simulink model "sop_codegen"  (R2024b)
settings: Solver=FixedStepAuto  StartTime=0.0  StopTime=inf  FixedStep=sopk_stepSize  RelTol=1e-3  SampleTimeConstraint=STIndependent  EnableMultiTasking=on
undefined symbols (not defined in the file): bmsc_CellMaxVolt, bmsc_CellMinVolt, bmsc_InternalChgResistX, bmsc_InternalChgResistY, bmsc_InternalChgResistZ, bmsc_InternalDischgResistX, bmsc_InternalDischgResistY, bmsc_InternalDischgResistZ, bmsc_NumberInPara, bmsc_NumberInSeries, sopc_ChargeDerate, sopc_ChgFaultDerate, sopc_DischargeDerate, sopc_DischgFaultDerate, sopc_SOCVsOCVX, sopc_SOCVsOCVY
settings Model: Creator=favv5g  LastModifiedBy=voillat
settings ConfigSet: Description=OpenECU configuration set for code generation under RTW-EC.
settings SolverCC: AlgebraicLoopSolver=TrustRegion  PositivePriorityOrder=on
settings DataIOCC: LimitDataPoints=on  SaveFormat=Array  SignalLoggingSaveFormat=ModelDataLogs
settings OptimizationCC: DefaultParameterBehavior=Inlined  InlineInvariantSignals=on  ExpressionDepthLimit=2147483647  StateBitsets=on  DataBitsets=on  ZeroExternalMemoryAtStartup=off  ZeroInternalMemoryAtStartup=off  NoFixptDivByZeroProtection=on  EfficientFloat2IntCast=on  LifeSpan=1  EfficientTunableParamExpr=on
settings DebuggingCC: SaveWithParameterizedLinksMsg=none  SignalResolutionControl=TryResolveAllWithWarning  MultiTaskDSMMsg=warning  MultiTaskCondExecSysMsg=none  SingleTaskRateTransMsg=error  CheckMatrixSingularityMsg=warning  VectorMatrixConversionMsg=warning  SignalLabelMismatchMsg=warning  UnconnectedInputMsg=warning  UnconnectedOutputMsg=warning  UnconnectedLineMsg=warning  AllowSymbolicDim=off  StateNameClashWarn=warning  SFUnexpectedBacktrackingDiag=warning  SFNoUnconditionalDefaultTransitionDiag=warning  SFExecutionAtInitializationDiag=none  ArithmeticOperatorsInVariantConditions=warning
settings HardwareCC: ProdBitPerPointer=32  ProdBitPerSizeT=32  ProdBitPerPtrDiffT=32  ProdLargestAtomicInteger=Long  ProdLargestAtomicFloat=Double  ProdEndianess=BigEndian  ProdWordSize=32  ProdHWDeviceType=Freescale->32-bit PowerPC  TargetIntDivRoundTo=Zero  TargetEndianess=BigEndian  TargetHWDeviceType=Freescale->32-bit PowerPC  ProdEqTarget=off
settings ModelReferenceCC: EnableRefExpFcnMdlSchedulingChecks=on  PropagateSignalLabelsOutOfModel=off
settings SFSimCC: SimUseLocalCustomCode=off  MATLABDynamicMemAlloc=off  CustomCodeUndefinedFunction=UseInterfaceOnly
settings RTWCC: Description=OpenECU Platform Target (ERT, optimised floating-point code)  SystemTargetFile=openecu_ert.tlc  MakeCommand=make_rtw optimized_floating_point=1  TemplateMakefile=openecu_ert_r2015b_64.tmf  RetainRTWFile=on  RTWUseLocalCustomCode=off  IncludeHyperlinkInReport=on  GPUComputeCapability=3.5
settings CodeAppCC: ForceParamTrailComments=on  IgnoreCustomStorageClasses=off  SimulinkDataObjDesc=on  CustomSymbolStrType=$N$R$M  InsertBlockDesc=on  StateflowObjectComments=on  InternalIdentifier=Classic
settings STFCustomTargetCC: TargetLibSuffix=.a  GenerateSampleERTMain=on  IncludeMdlTerminateFcn=off  CombineOutputUpdateFcns=on  IncludeFileDelimiter=UseQuote  ERTCustomFileBanners=on  SupportContinuousTime=off  RemoveResetFunc=on  MATLABClassNameForMDSCustomization=Simulink.SoftwareTarget.ERTCustomization  SystemTargetFile=openecu_ert.tlc
settings ERTTargetCC: MultiwordLength=2048  GenerateSampleERTMain=on  ParMdlRefBuildCompliant=off  CompOptLevelCompliant=off  ConcurrentExecutionCompliant=off  IncludeMdlTerminateFcn=off  IncludeFileDelimiter=UseQuote  SupportNonInlinedSFcns=on  ModelStepFunctionPrototypeControlCompliant=off  CPPClassGenCompliant=off  UseToolchainInfoCompliant=off  ExtModeMexFile=noextcomm  ERTSrcFileBannerTemplate=oe_code_c_template.cgt  ERTHdrFileBannerTemplate=oe_code_h_template.cgt  ERTDataSrcFileTemplate=oe_data_c_template.cgt  ERTDataHdrFileTemplate=oe_data_h_template.cgt  ERTCustomFileTemplate=example_file_process.tlc  GlobalDataDefinition=InSeparateSourceFile  GlobalDataReference=InSeparateHeaderFile  ConvertIfToSwitch=off  SuppressUnreachableDefaultCases=off  EnableUserReplacementTypes=on  DynamicArrayContainerType=coder::array
settings ConfigComp: CovMetricSettings=dw  CovSaveCumulativeToWorkspaceVar=on  CovSaveSingleToWorkspaceVar=on  CovExternalEMLEnable=off

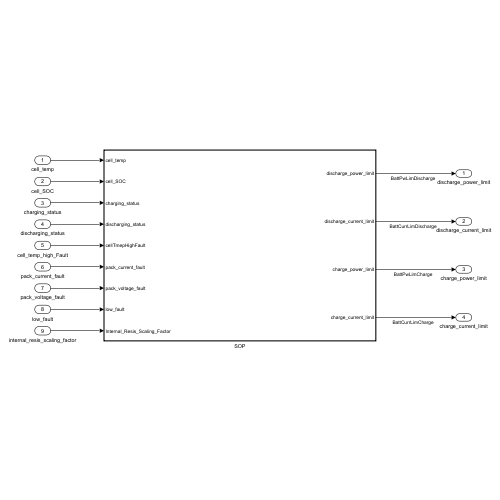
[thumbnail: Simulink's stored preview of the top-level diagram]
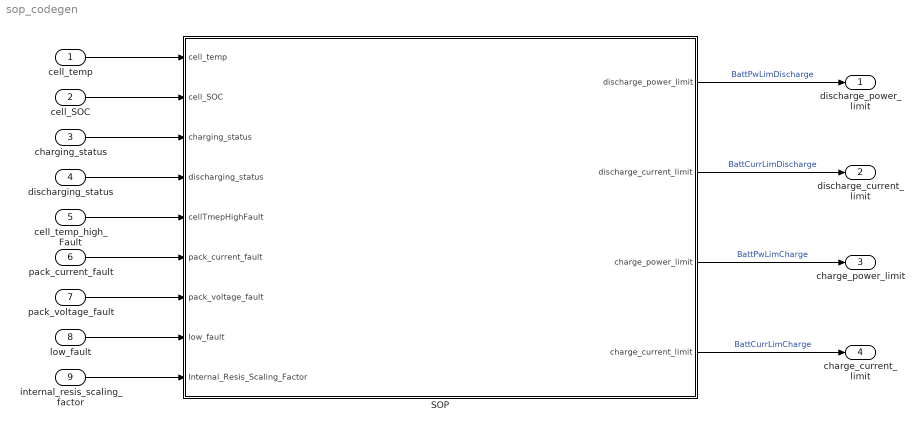
== system sop_codegen ==
  cell_temp : Inport  PortDimensions=40
  cell_SOC : Inport  Port=2  PortDimensions=40
  charging_status : Inport  Port=3
  discharging_status : Inport  Port=4
  cell_temp_high_Fault : Inport  Port=5
  pack_current_fault : Inport  Port=6
  pack_voltage_fault : Inport  Port=7
  low_fault : Inport  Port=8
  internal_resis_scaling_factor : Inport  Port=9  PortDimensions=40
  SOP : Subsystem  TreatAsAtomicUnit=on
  discharge_power_limit : Outport
  discharge_current_limit : Outport  Port=2
  charge_power_limit : Outport  Port=3
  charge_current_limit : Outport  Port=4
  wires:
  cell_temp/1 -> SOP/1(cell_temp)
  cell_SOC/1 -> SOP/2(cell_SOC)
  charging_status/1 -> SOP/3(charging_status)
  discharging_status/1 -> SOP/4(discharging_status)
  cell_temp_high_Fault/1 -> SOP/5(cellTmepHighFault)
  pack_current_fault/1 -> SOP/6(pack_current_fault)
  pack_voltage_fault/1 -> SOP/7(pack_voltage_fault)
  internal_resis_scaling_factor/1 -> SOP/9(Internal_Resis_Scaling_Factor)
  SOP/1(discharge_power_limit) -> discharge_power_limit/1  "BattPwLimDischarge"
  SOP/2(discharge_current_limit) -> discharge_current_limit/1  "BattCurrLimDischarge"
  SOP/3(charge_power_limit) -> charge_power_limit/1  "BattPwLimCharge"
  SOP/4(charge_current_limit) -> charge_current_limit/1  "BattCurrLimCharge"
  low_fault/1 -> SOP/8(low_fault)

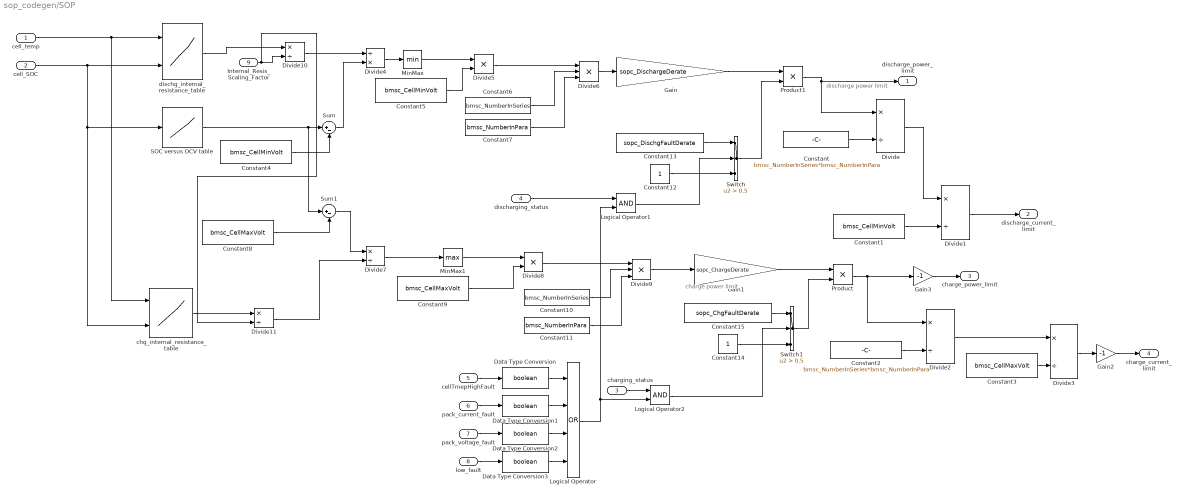
== system sop_codegen/SOP ==
  note: charge power limit
  note: discharge power limit
  cell_temp : Inport
  cell_SOC : Inport  Port=2
  charging_status : Inport  Port=3
  discharging_status : Inport  Port=4
  cellTmepHighFault : Inport  Port=5  OutDataTypeStr=uint8
  pack_current_fault : Inport  Port=6  OutDataTypeStr=uint8
  pack_voltage_fault : Inport  Port=7  OutDataTypeStr=uint8
  low_fault : Inport  Port=8  OutDataTypeStr=uint8
  Internal_Resis_Scaling_Factor : Inport  Port=9
  Constant : Constant  Value=bmsc_NumberInSeries*bmsc_NumberInPara
  Constant1 : Constant  Value=bmsc_CellMinVolt
  Constant10 : Constant  Value=bmsc_NumberInSeries
  Constant11 : Constant  Value=bmsc_NumberInPara
  Constant12 : Constant
  Constant13 : Constant  Value=sopc_DischgFaultDerate
  Constant14 : Constant
  Constant15 : Constant  Value=sopc_ChgFaultDerate
  Constant2 : Constant  Value=bmsc_NumberInSeries*bmsc_NumberInPara
  Constant3 : Constant  Value=bmsc_CellMaxVolt
  Constant4 : Constant  Value=bmsc_CellMinVolt
  Constant5 : Constant  Value=bmsc_CellMinVolt
  Constant6 : Constant  Value=bmsc_NumberInSeries
  Constant7 : Constant  Value=bmsc_NumberInPara
  Constant8 : Constant  Value=bmsc_CellMaxVolt
  Constant9 : Constant  Value=bmsc_CellMaxVolt
  Data Type Conversion{,1..3} (4 alike) : DataTypeConversion  OutDataTypeStr=boolean  SaturateOnIntegerOverflow=off  RndMeth=Floor
  Divide{,1..3,7,10..11} (7 alike) : Product  Inputs=*/
  Divide4 : Product  Inputs=/*
  Divide5 : Product  Inputs=**
  Divide6 : Product  Inputs=***
  Divide8 : Product  Inputs=**
  Divide9 : Product  Inputs=***
  Gain : Gain  Gain=sopc_DischargeDerate
  Gain1 : Gain  Gain=sopc_ChargeDerate
  Gain2 : Gain  Gain=-1
  Gain3 : Gain  Gain=-1
  Logical Operator : Logic  Operator=OR  Inputs=4  AllPortsSameDT=off  OutDataTypeStr=boolean
  Logical Operator1 : Logic  AllPortsSameDT=off  OutDataTypeStr=boolean
  Logical Operator2 : Logic  AllPortsSameDT=off  OutDataTypeStr=boolean
  MinMax : MinMax
  MinMax1 : MinMax  Function=max
  Product : Product
  Product1 : Product
  SOC versus OCV table : Lookup_n-D  NumberOfTableDimensions=1  BreakpointsForDimension1=sopc_SOCVsOCVX  Table=sopc_SOCVsOCVY  InternalRulePriority=Speed  RndMeth=Simplest
  Sum : Sum  Inputs=|+-
  Sum1 : Sum  Inputs=|+-
  Switch : Switch  Criteria=u2 > Threshold  Threshold=0.5  SaturateOnIntegerOverflow=off  InputSameDT=off
  Switch1 : Switch  Criteria=u2 > Threshold  Threshold=0.5  SaturateOnIntegerOverflow=off  InputSameDT=off
  chg_internal_resistance_table : Lookup_n-D  BreakpointsForDimension1=bmsc_InternalChgResistX  BreakpointsForDimension2=bmsc_InternalChgResistY  Table=bmsc_InternalChgResistZ  RndMeth=Simplest
      settings: InputPortMap=u0,u1
  dischg_internal_resistance_table : Lookup_n-D  BreakpointsForDimension1=bmsc_InternalDischgResistX  BreakpointsForDimension2=bmsc_InternalDischgResistY  Table=bmsc_InternalDischgResistZ  RndMeth=Simplest
      settings: InputPortMap=u0,u1
  discharge_power_limit : Outport
  discharge_current_limit : Outport  Port=2
  charge_power_limit : Outport  Port=3
  charge_current_limit : Outport  Port=4
  wires:
  Constant1/1 -> Divide1/2
  Constant2/1 -> Divide2/2
  Divide/1 -> Divide1/1
  Constant/1 -> Divide/2
  cell_temp/1 -> chg_internal_resistance_table/1, dischg_internal_resistance_table/1
  Divide1/1 -> discharge_current_limit/1
  Constant10/1 -> Divide9/2
  Divide9/1 -> Gain1/1
  Constant4/1 -> Sum/2
  Constant5/1 -> Divide5/2
  Constant7/1 -> Divide6/3
  Sum/1 -> Divide4/2
  Constant9/1 -> Divide8/2
  Divide3/1 -> Gain2/1
  SOC versus OCV table/1 -> Sum1/1, Sum/1
  Divide2/1 -> Divide3/1
  cell_SOC/1 -> SOC versus OCV table/1, chg_internal_resistance_table/2, dischg_internal_resistance_table/2
  Divide7/1 -> MinMax1/1
  MinMax1/1 -> Divide8/1
  Sum1/1 -> Divide7/1
  Divide6/1 -> Gain/1
  Divide4/1 -> MinMax/1
  Divide8/1 -> Divide9/1
  Constant8/1 -> Sum1/2
  Divide5/1 -> Divide6/1
  MinMax/1 -> Divide5/1
  Constant11/1 -> Divide9/3
  Constant6/1 -> Divide6/2
  Constant3/1 -> Divide3/2
  cellTmepHighFault/1 -> Data Type Conversion/1
  pack_current_fault/1 -> Data Type Conversion1/1
  pack_voltage_fault/1 -> Data Type Conversion2/1
  Constant12/1 -> Switch/3
  Constant13/1 -> Switch/1
  Logical Operator/1 -> Logical Operator2/2, Logical Operator1/2
  Constant14/1 -> Switch1/3
  Constant15/1 -> Switch1/1
  discharging_status/1 -> Logical Operator1/1
  Logical Operator1/1 -> Switch/2
  charging_status/1 -> Logical Operator2/1
  Logical Operator2/1 -> Switch1/2
  Switch1/1 -> Product/2
  Gain1/1 -> Product/1
  Product/1 -> Gain3/1, Divide2/1
  Switch/1 -> Product1/2
  Gain/1 -> Product1/1
  Product1/1 -> discharge_power_limit/1, Divide/1
  dischg_internal_resistance_table/1 -> Divide10/1
  Divide10/1 -> Divide4/1
  Internal_Resis_Scaling_Factor/1 -> Divide11/2, Divide10/2
  chg_internal_resistance_table/1 -> Divide11/1
  Divide11/1 -> Divide7/2
  Data Type Conversion/1 -> Logical Operator/1
  Data Type Conversion1/1 -> Logical Operator/2
  Data Type Conversion2/1 -> Logical Operator/3
  Data Type Conversion3/1 -> Logical Operator/4
  low_fault/1 -> Data Type Conversion3/1
  Gain2/1 -> charge_current_limit/1
  Gain3/1 -> charge_power_limit/1
